simulink model "SolarSailOld"  (R2024a)
settings: Solver=VariableStepAuto  StartTime=0.0  StopTime=60*120  RelTol=1e-3
model workspace (MAT data in the model file):
  LocalBodyOffset = [45 0 0]
undefined symbols (not defined in the file): juliandate, magnitude
libraries: aerolibutil x12, matrix_library x8, aerolibconvert2 x4, sharedtransform x4, slpidlib x2, simulink_extras x2, aerolibsatdyn x1, aerolibobsolete x1, aerolibattitudesys x1, simulink x1, vrlib x1
(part 2 of 2)

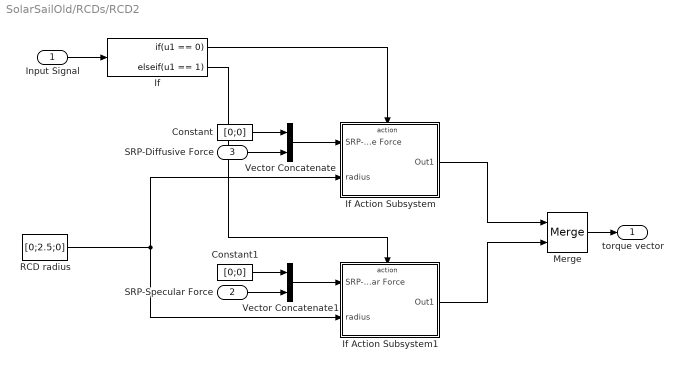
== system SolarSailOld/RCDs/RCD2 ==
  Input Signal : Inport
  SRP-Specular Force : Inport  Port=2
  SRP-Diffusive Force : Inport  Port=3
  Constant : Constant  Value=[0;0]
  Constant1 : Constant  Value=[0;0]
  If : If  IfExpression=u1 == 0  ElseIfExpressions=u1 == 1  ShowElse=off
  If Action Subsystem : Subsystem  TreatAsAtomicUnit=on
  If Action Subsystem1 : Subsystem  TreatAsAtomicUnit=on
  Merge : Merge
  RCD radius : Constant  Value=[0;2.5;0]
  Vector Concatenate : Concatenate
  Vector Concatenate1 : Concatenate
  torque vector : Outport
  wires:
  Input Signal/1 -> If/1
  If/1 -> If Action Subsystem/Action
  Merge/1 -> torque vector/1
  If Action Subsystem/1(Out1) -> Merge/1
  If/2 -> If Action Subsystem1/Action
  If Action Subsystem1/1(Out1) -> Merge/2
  RCD radius/1 -> If Action Subsystem/2(radius), If Action Subsystem1/2(radius)
  Vector Concatenate/1 -> If Action Subsystem/1(SRP-Diffusive Force)
  Constant/1 -> Vector Concatenate/1
  SRP-Diffusive Force/1 -> Vector Concatenate/2
  SRP-Specular Force/1 -> Vector Concatenate1/2
  Constant1/1 -> Vector Concatenate1/1
  Vector Concatenate1/1 -> If Action Subsystem1/1(SRP-Specular Force)

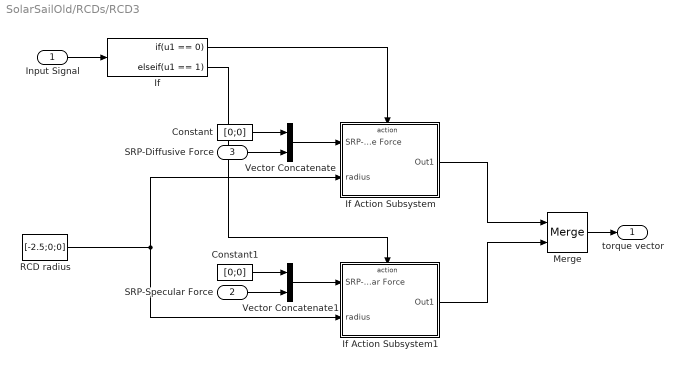
== system SolarSailOld/RCDs/RCD3 ==
  Input Signal : Inport
  SRP-Specular Force : Inport  Port=2
  SRP-Diffusive Force : Inport  Port=3
  Constant : Constant  Value=[0;0]
  Constant1 : Constant  Value=[0;0]
  If : If  IfExpression=u1 == 0  ElseIfExpressions=u1 == 1  ShowElse=off
  If Action Subsystem : Subsystem  TreatAsAtomicUnit=on
  If Action Subsystem1 : Subsystem  TreatAsAtomicUnit=on
  Merge : Merge
  RCD radius : Constant  Value=[-2.5;0;0]
  Vector Concatenate : Concatenate
  Vector Concatenate1 : Concatenate
  torque vector : Outport
  wires:
  Input Signal/1 -> If/1
  If/1 -> If Action Subsystem/Action
  Merge/1 -> torque vector/1
  If Action Subsystem/1(Out1) -> Merge/1
  If/2 -> If Action Subsystem1/Action
  If Action Subsystem1/1(Out1) -> Merge/2
  RCD radius/1 -> If Action Subsystem/2(radius), If Action Subsystem1/2(radius)
  Vector Concatenate/1 -> If Action Subsystem/1(SRP-Diffusive Force)
  Constant/1 -> Vector Concatenate/1
  SRP-Diffusive Force/1 -> Vector Concatenate/2
  SRP-Specular Force/1 -> Vector Concatenate1/2
  Constant1/1 -> Vector Concatenate1/1
  Vector Concatenate1/1 -> If Action Subsystem1/1(SRP-Specular Force)

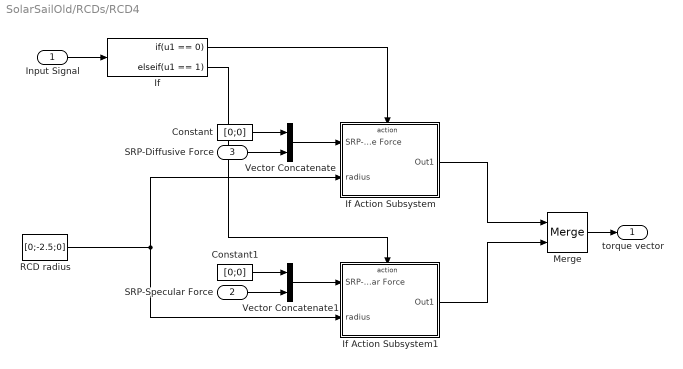
== system SolarSailOld/RCDs/RCD4 ==
  Input Signal : Inport
  SRP-Specular Force : Inport  Port=2
  SRP-Diffusive Force : Inport  Port=3
  Constant : Constant  Value=[0;0]
  Constant1 : Constant  Value=[0;0]
  If : If  IfExpression=u1 == 0  ElseIfExpressions=u1 == 1  ShowElse=off
  If Action Subsystem : Subsystem  TreatAsAtomicUnit=on
  If Action Subsystem1 : Subsystem  TreatAsAtomicUnit=on
  Merge : Merge
  RCD radius : Constant  Value=[0;-2.5;0]
  Vector Concatenate : Concatenate
  Vector Concatenate1 : Concatenate
  torque vector : Outport
  wires:
  Input Signal/1 -> If/1
  If/1 -> If Action Subsystem/Action
  Merge/1 -> torque vector/1
  If Action Subsystem/1(Out1) -> Merge/1
  If/2 -> If Action Subsystem1/Action
  If Action Subsystem1/1(Out1) -> Merge/2
  RCD radius/1 -> If Action Subsystem/2(radius), If Action Subsystem1/2(radius)
  Vector Concatenate/1 -> If Action Subsystem/1(SRP-Diffusive Force)
  Constant/1 -> Vector Concatenate/1
  SRP-Diffusive Force/1 -> Vector Concatenate/2
  SRP-Specular Force/1 -> Vector Concatenate1/2
  Constant1/1 -> Vector Concatenate1/1
  Vector Concatenate1/1 -> If Action Subsystem1/1(SRP-Specular Force)

== system SolarSailOld/SRP Force Model/Multiplication ==
  SRP : Inport
  Sun Angle : Inport  Port=2
  Area : Inport  Port=3
  Cos : Trigonometry  Operator=cos
  Gain : Gain  Gain=2
  Product : Product  Inputs=3
  Scope : Scope
  Square : Math  Operator=square
  SRP Force : Outport
  wires:
  Product/1 -> Gain/1
  SRP/1 -> Product/1
  Area/1 -> Product/2
  Cos/1 -> Square/1
  Sun Angle/1 -> Cos/1
  Square/1 -> Product/3
  Gain/1 -> SRP Force/1

== system SolarSailOld/CubeSat Animation/Antenna Position to VRML/ECEF to VRML ==
  M : Inport  PortDimensions=3
  Selector : Selector  InputPortWidth=3  IndexOptions=Index vector (dialog)  Indices=[2 3 1]  OutputSizes=1
  VR : Outport  PortDimensions=3  VectorParamsAs1DForOutWhenUnconnected=off
  wires:
  M/1 -> Selector/1
  Selector/1 -> VR/1

== system SolarSailOld/CubeSat Animation/Compute Earth Rotation Rate/Quaternion to VRML ==
  q : Inport
  Demux : Demux
  Gain : Gain  Gain=2
  Gain3 : Gain  Gain=[-1 1 1 1]
  Mux : Mux
  Selector : Selector  InputPortWidth=4  IndexOptions=Index vector (dialog)  Indices=[2 4 3 1]  OutputSizes=1
  Trigonometric Function : Trigonometry  Operator=acos
  AxisAngle : Outport  VectorParamsAs1DForOutWhenUnconnected=off
  wires:
  Demux/1 -> Trigonometric Function/1
  Trigonometric Function/1 -> Gain/1
  Mux/1 -> Selector/1
  q/1 -> Demux/1
  Gain3/1 -> AxisAngle/1
  Selector/1 -> Gain3/1
  Gain/1 -> Mux/1
  Demux/2 -> Mux/2
  Demux/3 -> Mux/3
  Demux/4 -> Mux/4

== system SolarSailOld/CubeSat Animation/Compute Umbra Translation/unitVec ==
  I : Inport
  Divide : Product  Inputs=*/
  Dot Product : DotProduct  OutDataTypeStr=Inherit: Inherit via internal rule
  Sqrt : Sqrt
  O : Outport  VectorParamsAs1DForOutWhenUnconnected=off
  wires:
  Dot Product/1 -> Sqrt/1
  I/1 -> Divide/1, Dot Product/1, Dot Product/2
  Divide/1 -> O/1
  Sqrt/1 -> Divide/2

== system SolarSailOld/CubeSat Animation/Sat Position to VRML/ECEF to VRML ==
  M : Inport  PortDimensions=3
  Selector : Selector  InputPortWidth=3  IndexOptions=Index vector (dialog)  Indices=[2 3 1]  OutputSizes=1
  VR : Outport  PortDimensions=3  VectorParamsAs1DForOutWhenUnconnected=off
  wires:
  M/1 -> Selector/1
  Selector/1 -> VR/1

== system SolarSailOld/CubeSat Animation/Sun Position to VRML/ECEF to VRML ==
  M : Inport  PortDimensions=3
  Selector : Selector  InputPortWidth=3  IndexOptions=Index vector (dialog)  Indices=[2 3 1]  OutputSizes=1
  VR : Outport  PortDimensions=3  VectorParamsAs1DForOutWhenUnconnected=off
  wires:
  M/1 -> Selector/1
  Selector/1 -> VR/1

== system SolarSailOld/RCDs/RCD1/If Action Subsystem ==
  SRP-Diffusive Force : Inport
  radius : Inport  Port=2
  Action Port : ActionPort  ActionPortLabel=if(u1 == 0)
  Cross Product : matrix_library/Cross Product
  Out1 : Outport
  wires:
  Cross Product/1 -> Out1/1
  SRP-Diffusive Force/1 -> Cross Product/2
  radius/1 -> Cross Product/1

== system SolarSailOld/RCDs/RCD1/If Action Subsystem1 ==
  SRP-Specular Force : Inport
  radius : Inport  Port=2
  Action Port : ActionPort  ActionPortLabel=elseif(u1 == 1)
  Cross Product : matrix_library/Cross Product
  Out1 : Outport
  wires:
  Cross Product/1 -> Out1/1
  SRP-Specular Force/1 -> Cross Product/2
  radius/1 -> Cross Product/1

== system SolarSailOld/RCDs/RCD2/If Action Subsystem ==
  SRP-Diffusive Force : Inport
  radius : Inport  Port=2
  Action Port : ActionPort  ActionPortLabel=if(u1 == 0)
  Cross Product : matrix_library/Cross Product
  Out1 : Outport
  wires:
  Cross Product/1 -> Out1/1
  SRP-Diffusive Force/1 -> Cross Product/2
  radius/1 -> Cross Product/1

== system SolarSailOld/RCDs/RCD2/If Action Subsystem1 ==
  SRP-Specular Force : Inport
  radius : Inport  Port=2
  Action Port : ActionPort  ActionPortLabel=elseif(u1 == 1)
  Cross Product : matrix_library/Cross Product
  Out1 : Outport
  wires:
  Cross Product/1 -> Out1/1
  SRP-Specular Force/1 -> Cross Product/2
  radius/1 -> Cross Product/1

== system SolarSailOld/RCDs/RCD3/If Action Subsystem ==
  SRP-Diffusive Force : Inport
  radius : Inport  Port=2
  Action Port : ActionPort  ActionPortLabel=if(u1 == 0)
  Cross Product : matrix_library/Cross Product
  Out1 : Outport
  wires:
  Cross Product/1 -> Out1/1
  SRP-Diffusive Force/1 -> Cross Product/2
  radius/1 -> Cross Product/1

== system SolarSailOld/RCDs/RCD3/If Action Subsystem1 ==
  SRP-Specular Force : Inport
  radius : Inport  Port=2
  Action Port : ActionPort  ActionPortLabel=elseif(u1 == 1)
  Cross Product : matrix_library/Cross Product
  Out1 : Outport
  wires:
  Cross Product/1 -> Out1/1
  SRP-Specular Force/1 -> Cross Product/2
  radius/1 -> Cross Product/1

== system SolarSailOld/RCDs/RCD4/If Action Subsystem ==
  SRP-Diffusive Force : Inport
  radius : Inport  Port=2
  Action Port : ActionPort  ActionPortLabel=if(u1 == 0)
  Cross Product : matrix_library/Cross Product
  Out1 : Outport
  wires:
  Cross Product/1 -> Out1/1
  SRP-Diffusive Force/1 -> Cross Product/2
  radius/1 -> Cross Product/1

== system SolarSailOld/RCDs/RCD4/If Action Subsystem1 ==
  SRP-Specular Force : Inport
  radius : Inport  Port=2
  Action Port : ActionPort  ActionPortLabel=elseif(u1 == 1)
  Cross Product : matrix_library/Cross Product
  Out1 : Outport
  wires:
  Cross Product/1 -> Out1/1
  SRP-Specular Force/1 -> Cross Product/2
  radius/1 -> Cross Product/1

== matlab function SolarSailOld/Sun Angle1/Quat2RotMat ==
  data: quat input; rotm output
function rotm = fcn(quat)
rotm = quat2rotm(quat');

== matlab function SolarSailOld/Sun Angle1/sun_position ==
  data: julian_date input; r_sun output
function r_sun = sun_position(julian_date)
    % Compute the Sun's position in ECI coordinates (in km)
    % 'julian_date' is the current time in Julian date format.
    
    % Declare the planetEphemeris function as extrinsic to prevent code generation
    coder.extrinsic('planetEphemeris');

    % Use planetEphemeris from Aerospace Toolbox
    r_sun = [0,0,0];
    r_sun = planetEphemeris(julian_date, 'Earth', 'Sun');
end

== matlab function SolarSailOld/SRP Force Model/Quat2RotMat ==
  data: quat input; rotm output
function rotm = fcn(quat)
rotm = quat2rotm(quat');

== matlab function SolarSailOld/MATLAB Function ==
  data: quat input; eulerAngles output
function eulerAngles = fcn(quat)
eulerAngles = quat2eul(quat');

== matlab function SolarSailOld/Reaction Wheel/Torque Limiter ==
  data: desired_T input; T output; limit input
function T = limiter(desired_T, limit)

if (desired_T > limit)
    T = limit;
elseif (desired_T < -limit)
    T = -limit;
else
    T = desired_T;
end

== matlab function SolarSailOld/icrf2lvlh/MATLAB Function ==
  data: pos input; DCM output; vel input
function DCM = DCM_icrf2lvlh(pos,vel)

% Find unit vectors for creating DCM
X_hat = pos/vecnorm(pos); % direction of position vector
h = cross(pos,vel); 
Z_hat = h/vecnorm(h); % direction of + orbit normal
Y_hat = cross(Z_hat,X_hat); % direction of velocity 
Y_hat = Y_hat/vecnorm(Y_hat); % double check normalize

DCM = [X_hat, Y_hat, Z_hat];

% https://space.stackexchange.com/questions/33803/eci-to-lvlh-conversion

== matlab function SolarSailOld/RCD Converter/MATLAB Function ==
  data: RCD2 output; RCD4 output; T_x input; T_on input; T_off input; prevRCD2 input; prevRCD4 input
function [RCD2,RCD4] = fcn(T_x, T_on, T_off, prevRCD2, prevRCD4)

if (T_x > T_on)
    % Turn one side on
    RCD2 = 1;
    RCD4 = 0;
elseif (T_x < -T_on)
    % Turn other side on
    RCD2 = 0;
    RCD4 = 1;
elseif (T_x < T_off && T_x > -T_off)
    % Turn both off
    RCD2 = 0;
    RCD4 = 0;
else 
    % Don't change
    RCD2 = prevRCD2;
    RCD4 = prevRCD4;
end

== matlab function SolarSailOld/RCD Converter/MATLAB Function1 ==
  data: RCD1 output; RCD3 output; T_y input; T_on input; T_off input; reset1 output; reset3 output
function [RCD1,RCD3, reset1, reset3] = fcn(T_y, T_on, T_off)

if (T_y > T_on)
    % Turn one side on
    RCD1 = false;
    RCD3 = true;
    reset1 = true;
    reset3 = false;
elseif (T_y < -T_on)
    % Turn other side on
    RCD1 = true;
    RCD3 = false;
    reset1 = false;
    reset3 = true;
elseif (T_y < T_off && T_y > -T_off)
    % Turn both off
    RCD1 = false;
    RCD3 = false;
    reset1 = true;
    reset3 = true;
else
    % Keep same state
    RCD1 = false;
    RCD3 = false;
    reset1 = false;
    reset3 = false;
end

== matlab function SolarSailOld/Sun Angle/MATLAB Function ==
  data: sunAngle output; N_icrf input; r_satsun input
function sunAngle = fcn(N_icrf, r_satsun)

S_hat = r_satsun / vecnorm(r_satsun);
N_hat = N_icrf / vecnorm(N_icrf);

sunAngle = acos(dot(S_hat,N_hat));

== matlab function SolarSailOld/Sun Angle/Quat2RotMat ==
  data: quat input; rotm output
function rotm = fcn(quat)
rotm = quat2rotm(quat');

== matlab function SolarSailOld/Sun Angle/sun_position ==
  data: julian_date input; r_sun output
function r_sun = sun_position(julian_date)
    % Compute the Sun's position in ECI coordinates (in km)
    % 'julian_date' is the current time in Julian date format.
    
    % Declare the planetEphemeris function as extrinsic to prevent code generation
    coder.extrinsic('planetEphemeris');

    % Use planetEphemeris from Aerospace Toolbox
    r_sun = [0,0,0];
    r_sun = planetEphemeris(julian_date, 'Earth', 'Sun');
end
